simulink model "CarE_Model"  (R2019b)
settings: Solver=VariableStepAuto  StartTime=0.0  StopTime=inf  RelTol=1e-3
(part 5 of 5)

== matlab function CarE_Model/CarE_System/Optimization_module/MATLAB Function ==
  data: SF_VH input; speed_suggestion output; SF_VC input; r input; max_speed input; a_vehicle input; event_id input; gravity input; avg_speed input; rate_acc input; rate_desacc input; crit_gap input; pos_ecar_x input; pos_ecar_z input; rot_ecar input; pos_lead_car_x input; pos_lead_car_z input; speed_lead_car input; olanecar_presence input; pos_olane_car_x input; pos_olane_car_z input; rot_olane_car input; speed_olane_car input; check_if_hit input; collisiondetection input; Mean_acc_road input; SD_acc_road input; acc_road_today input; road_surface_st input; road_cond_st input; weather_st input; time_day_st input; avgspeed_data input
function speed_suggestion=speed_suggest_Fun(SF_VH,SF_VC,r,max_speed,a_vehicle,event_id,gravity,avg_speed,rate_acc,rate_desacc,crit_gap,pos_ecar_x,pos_ecar_z,rot_ecar,pos_lead_car_x,pos_lead_car_z,speed_lead_car,olanecar_presence,pos_olane_car_x,pos_olane_car_z,rot_olane_car,speed_olane_car,check_if_hit,collisiondetection,Mean_acc_road,SD_acc_road,acc_road_today,road_surface_st,road_cond_st,weather_st,time_day_st,avgspeed_data) 
speed_suggestion=0;
 coder.extrinsic('Opt_Fun')

[speed_opt,max_fun]=Opt_Fun(SF_VH,SF_VC,r,max_speed,a_vehicle,event_id,gravity,avg_speed,rate_acc,rate_desacc,crit_gap,pos_ecar_x,pos_ecar_z,rot_ecar,pos_lead_car_x,pos_lead_car_z,speed_lead_car,olanecar_presence,pos_olane_car_x,pos_olane_car_z,rot_olane_car,speed_olane_car,check_if_hit,collisiondetection,Mean_acc_road,SD_acc_road,acc_road_today,road_surface_st,road_cond_st,weather_st,time_day_st,avgspeed_data); 
speed_suggestion=speed_opt*3.6;
end

== matlab function CarE_Model/CarE_System/MATLAB Function ==
  data: Health_factor input; HF_modified output; SF input
function HF_modified = Modify_HealthFactor(Health_factor,SF)

    %how close the HF is from the lowest point
    Dif=Health_factor-1;
    HF_modified=Health_factor-Dif*SF;

end

== matlab function CarE_Model/CarE_System/Output Module/Body_mapping/MATLAB Function ==
  data: anger input; cabine_st output; disgust input; fear input; happiness input; neutral input; sadness input; surprise input; tires_st output; wheels_st output; motor_st output; dashboard_st output; door_st output; body_st output; windshield_st output; ligths_st output; comm_st output; stress input
function [cabine_st,tires_st,wheels_st,motor_st,dashboard_st,door_st,body_st,windshield_st,ligths_st,comm_st] = body_map(anger,disgust,fear,happiness,neutral,sadness, surprise,stress)
    cabine_st=0;
    tires_st=0;
    wheels_st=0;
    motor_s=0;
    dashboard_st=0;
    door_st=0;
    body_st=0;
    windshield_st=0;
    ligths_st=0;
    comm_st=0;
     coder.extrinsic('bodymap')
    [cabine_st,tires_st,wheels_st,motor_st,dashboard_st,door_st,body_st,windshield_st,ligths_st,comm_st] = bodymapfn(anger,disgust,fear,happiness,neutral,sadness, surprise,stress);
end
